simulink model "snake_model"  (R2018a)
settings: Solver=FixedStepAuto  StartTime=0.0  StopTime=Tmax  FixedStep=0.001  RelTol=1e-3
values from neighbouring files (symbols this model uses):
  theta_max = min(theta_max, pi/2)    [find_sat.m]    (also in run_3D_simulation.m = find_sat(jointCtrl.shape, (snake.n-1)/2, jointCtrl.alpha))
undefined symbols (not defined in the file or in its folder): attCtrl, ctrlSettings, dragcoeff, guidance, jointCtrl, pp, snake, thrustAlloc, velCtrl, y_0
libraries: vrlib x1, sharedutil x1
settings Model: Creator=ilborlau  LastModifiedBy=12037

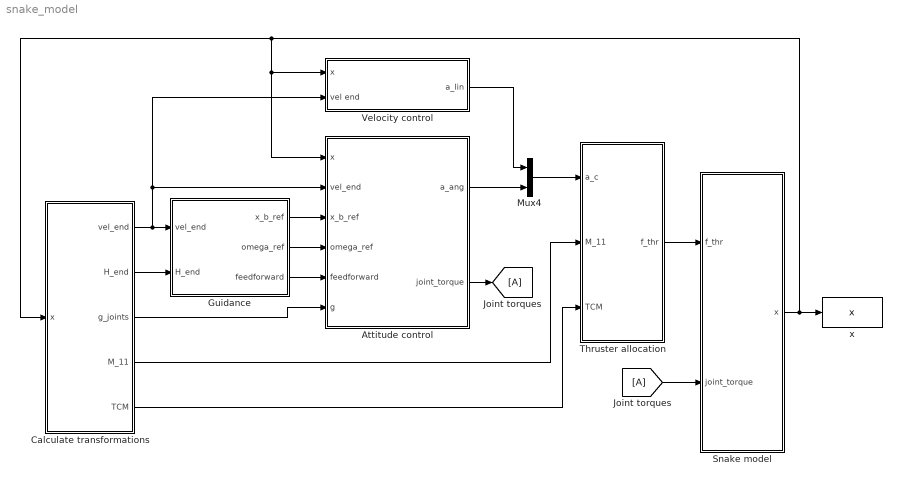
== system snake_model ==
  Attitude control : Subsystem
  Calculate transformations : Subsystem
  Guidance : Subsystem
  Mux4 : Mux  Inputs=2
  Snake model : Subsystem
  Thruster allocation : Subsystem
  Velocity control : Subsystem
  x : ToWorkspace  VariableName=x  SaveFormat=Structure With Time  SampleTime=-1
  wires:
  Guidance/1(x_b_ref) -> Attitude control/3(x_b_ref)
  [A] -> Snake model/2(joint_torque)
  Guidance/2(omega_ref) -> Attitude control/4(omega_ref)
  Guidance/3(feedforward) -> Attitude control/5(feedforward)
  Velocity control/1(a_lin) -> Mux4/1
  Attitude control/1("a_ang ") -> Mux4/2
  Calculate transformations/2(H_end) -> Guidance/2(H_end)
  Calculate transformations/1(vel_end) -> Guidance/1(vel_end), Velocity control/2(vel end), Attitude control/2(vel_end)
  Calculate transformations/5(TCM) -> Thruster allocation/3(TCM)
  Snake model/1(x) -> x/1, Calculate transformations/1(x), Velocity control/1(x), Attitude control/1(x)
  Thruster allocation/1(f_thr) -> Snake model/1(f_thr)
  Calculate transformations/4(M_11) -> Thruster allocation/2(M_11)
  Attitude control/2(joint_torque) -> [A]
  Calculate transformations/3(g_joints) -> Attitude control/6(g)
  Mux4/1 -> Thruster allocation/1(a_c)

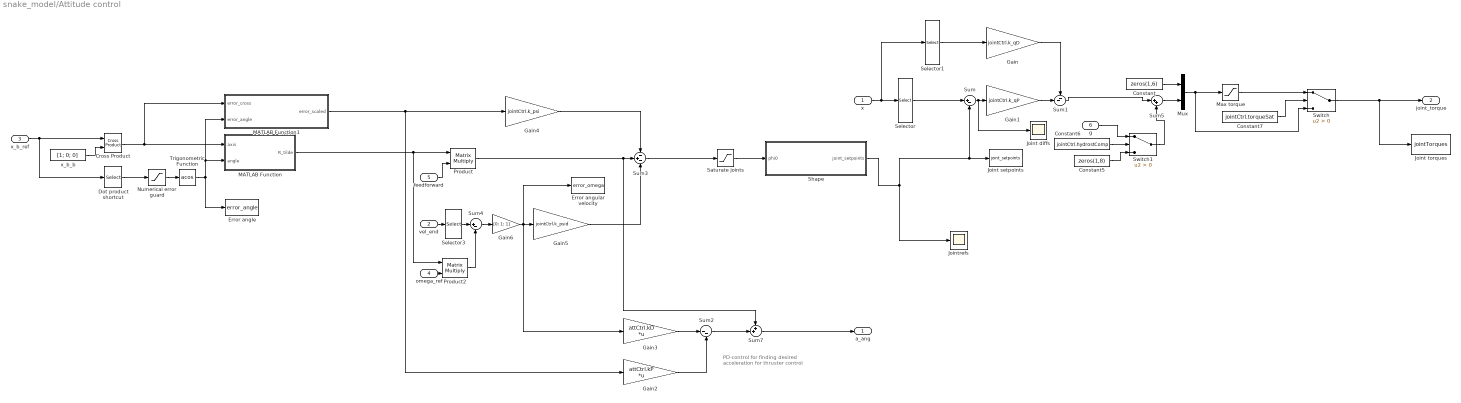
== system snake_model/Attitude control ==
  note: PD-control for finding desired acceleration for thruster control
  x : Inport
  vel_end : Inport  Port=2
  x_b_ref : Inport  Port=3
  omega_ref : Inport  Port=4
  feedforward : Inport  Port=5
  g : Inport  Port=6
  Constant : Constant  Value=zeros(1,6)
  Constant5 : Constant  Value=zeros(1,8)
  Constant6 : Constant  Value=jointCtrl.hydrostComp
  Constant7 : Constant  Value=jointCtrl.torqueSat
  Cross Product : vrlib/Utilities/Cross Product
      settings: SourceProductBaseCode=VR
  Dot product shortcut : Selector  InputPortWidth=3  IndexOptions=Index vector (dialog)  Indices=1  OutputSizes=1
  Error angle : ToWorkspace  VariableName=error_angle  SaveFormat=Structure With Time  SampleTime=-1
  Error angular velocity : ToWorkspace  VariableName=error_omega  SaveFormat=Structure With Time  SampleTime=-1
  Gain : Gain  Gain=jointCtrl.k_qD
  Gain1 : Gain  Gain=jointCtrl.k_qP
  Gain2 : Gain  Gain=attCtrl.kP  Multiplication=Matrix(K*u) (u vector)
  Gain3 : Gain  Gain=attCtrl.kD  Multiplication=Matrix(K*u) (u vector)
  Gain4 : Gain  Gain=jointCtrl.k_psi
  Gain5 : Gain  Gain=jointCtrl.k_psid
  Gain6 : Gain  Gain=[0; 1; 1]
  Joint diffs : Scope
  Joint setpoints : ToWorkspace  VariableName=joint_setpoints  SaveFormat=Structure With Time  SampleTime=-1
  Joint torques : ToWorkspace  VariableName=jointTorques  SaveFormat=Structure With Time  SampleTime=-1
  Jointrefs : Scope
  MATLAB Function : MATLAB Function  TreatAsAtomicUnit=on
  MATLAB Function1 : MATLAB Function  TreatAsAtomicUnit=on
  Max torque : Saturate  UpperLimit=11  LowerLimit=-11
  Mux : Mux  Inputs=2
  Numerical error guard : Saturate  UpperLimit=1  LowerLimit=-1
  Product : Product  Multiplication=Matrix(*)
  Product2 : Product  Multiplication=Matrix(*)
  Saturate joints : Saturate  UpperLimit=theta_max  LowerLimit=-theta_max
  Selector : Selector  InputPortWidth=11+2*snake.n  IndexOptions=Index vector (dialog)  Indices=8:6+snake.n  OutputSizes=1
  Selector1 : Selector  InputPortWidth=11+2*snake.n  IndexOptions=Index vector (dialog)  Indices=13+snake.n:11+2*snake.n  OutputSizes=1
  Selector3 : Selector  InputPortWidth=6  IndexOptions=Index vector (dialog)  Indices=4:6  OutputSizes=1
  Shape : MATLAB Function  TreatAsAtomicUnit=on
  Sum : Sum  Inputs=|+-
  Sum1 : Sum  Inputs=--|
  Sum2 : Sum  Inputs=|--
  Sum3 : Sum  Inputs=-+-
  Sum4 : Sum  Inputs=|+-
  Sum5 : Sum  Inputs=|++
  Sum7 : Sum  Inputs=++|
  Switch : Switch  Criteria=u2 > Threshold
  Switch1 : Switch  Criteria=u2 > Threshold
  Trigonometric Function : Trigonometry  Operator=acos
  x_b_b : Constant  Value=[1; 0; 0]
  "a_ang " : Outport
  joint_torque : Outport  Port=2
  wires:
  x_b_ref/1 -> Dot product shortcut/1, Cross Product/1
  omega_ref/1 -> Product2/2
  x/1 -> Selector1/1, Selector/1
  Sum/1 -> Joint diffs/1, Gain1/1
  Selector/1 -> Sum/1
  Gain1/1 -> Sum1/2
  Gain/1 -> Sum1/1
  Mux/1 -> Max torque/1, Switch/3
  Constant/1 -> Mux/1
  Shape/1(joint_setpoints) -> Sum/2, Joint setpoints/1, Jointrefs/1
  Gain3/1 -> Sum2/1
  Gain2/1 -> Sum2/2
  Sum2/1 -> Sum7/2
  x_b_b/1 -> Cross Product/2
  Cross Product/1 -> MATLAB Function/1(axis), MATLAB Function1/1(error_cross)
  vel_end/1 -> Selector3/1
  Selector3/1 -> Sum4/1
  MATLAB Function/1(R_tilde) -> Product/1, Product2/1
  feedforward/1 -> Product/2
  Sum4/1 -> Gain6/1
  Product2/1 -> Sum4/2
  Gain5/1 -> Sum3/3
  Gain4/1 -> Sum3/1
  Sum3/1 -> Saturate joints/1
  MATLAB Function1/1(error_scaled) -> Gain4/1, Gain2/1
  Selector1/1 -> Gain/1
  Dot product shortcut/1 -> Numerical error guard/1
  Numerical error guard/1 -> Trigonometric Function/1
  Trigonometric Function/1 -> Error angle/1, MATLAB Function1/2(error_angle), MATLAB Function/2(angle)
  Saturate joints/1 -> Shape/1(phi0)
  Switch/1 -> Joint torques/1, joint_torque/1
  Sum1/1 -> Sum5/1
  Sum7/1 -> "a_ang "/1
  Max torque/1 -> Switch/1
  Sum5/1 -> Mux/2
  Constant5/1 -> Switch1/3
  g/1 -> Switch1/1
  Constant6/1 -> Switch1/2
  Switch1/1 -> Sum5/2
  Constant7/1 -> Switch/2
  Product/1 -> Sum7/1, Sum3/2
  Gain6/1 -> Error angular velocity/1, Gain5/1, Gain3/1

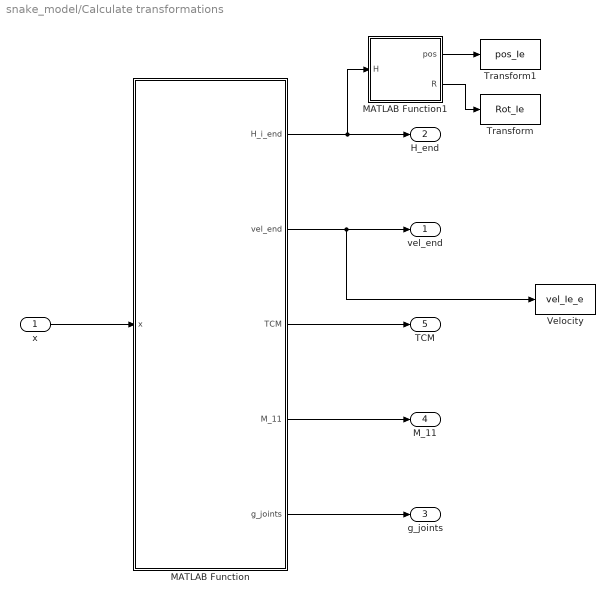
== system snake_model/Calculate transformations ==
  x : Inport
  MATLAB Function : MATLAB Function  TreatAsAtomicUnit=on
  MATLAB Function1 : MATLAB Function  TreatAsAtomicUnit=on
  Transform : ToWorkspace  VariableName=Rot_Ie  SaveFormat=Structure With Time  SampleTime=-1
  Transform1 : ToWorkspace  VariableName=pos_Ie  SaveFormat=Structure With Time  SampleTime=-1
  Velocity : ToWorkspace  VariableName=vel_Ie_e  SaveFormat=Structure With Time  SampleTime=-1
  vel_end : Outport
  H_end : Outport  Port=2
  g_joints : Outport  Port=3
  M_11 : Outport  Port=4
  TCM : Outport  Port=5
  wires:
  x/1 -> MATLAB Function/1(x)
  MATLAB Function/1(H_i_end) -> MATLAB Function1/1(H), H_end/1
  MATLAB Function/3(TCM) -> TCM/1
  MATLAB Function/2(vel_end) -> vel_end/1, Velocity/1
  MATLAB Function1/2(R) -> Transform/1
  MATLAB Function1/1(pos) -> Transform1/1
  MATLAB Function/5(g_joints) -> g_joints/1
  MATLAB Function/4(M_11) -> M_11/1

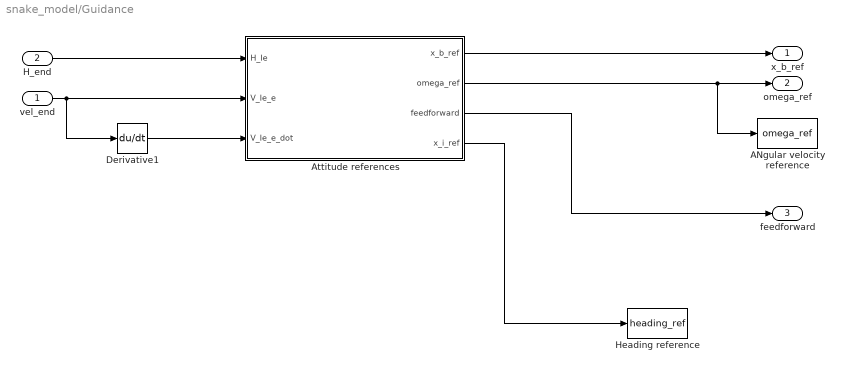
== system snake_model/Guidance ==
  vel_end : Inport
  H_end : Inport  Port=2
  ANgular velocity reference : ToWorkspace  VariableName=omega_ref  SaveFormat=Structure With Time  SampleTime=-1
  Attitude references : MATLAB Function  TreatAsAtomicUnit=on
  Derivative1 : Derivative  CoefficientInTFapproximation=1/15
  Heading reference : ToWorkspace  VariableName=heading_ref  SaveFormat=Structure With Time  SampleTime=-1
  x_b_ref : Outport
  omega_ref : Outport  Port=2
  feedforward : Outport  Port=3
  wires:
  H_end/1 -> Attitude references/1(H_Ie)
  Attitude references/1(x_b_ref) -> x_b_ref/1
  Attitude references/3(feedforward) -> feedforward/1
  Attitude references/4(x_i_ref) -> Heading reference/1
  vel_end/1 -> Derivative1/1, Attitude references/2(V_Ie_e)
  Attitude references/2(omega_ref) -> ANgular velocity reference/1, omega_ref/1
  Derivative1/1 -> Attitude references/3(V_Ie_e_dot)

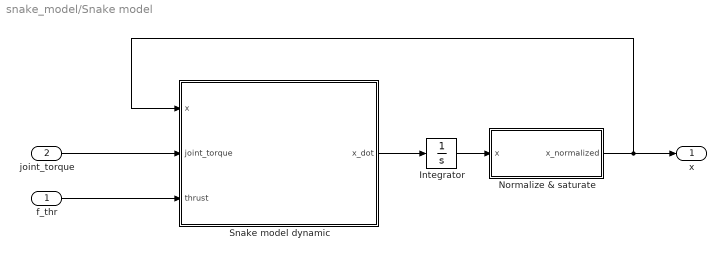
== system snake_model/Snake model ==
  f_thr : Inport
  joint_torque : Inport  Port=2
  Integrator : Integrator  InitialCondition=y_0
  Normalize & saturate : Subsystem
  Snake model dynamic : MATLAB Function  TreatAsAtomicUnit=on
  x : Outport
  wires:
  Snake model dynamic/1(x_dot) -> Integrator/1
  joint_torque/1 -> Snake model dynamic/2(joint_torque)
  f_thr/1 -> Snake model dynamic/3(thrust)
  Normalize & saturate/1(x_normalized) -> x/1, Snake model dynamic/1(x)
  Integrator/1 -> Normalize & saturate/1(x)

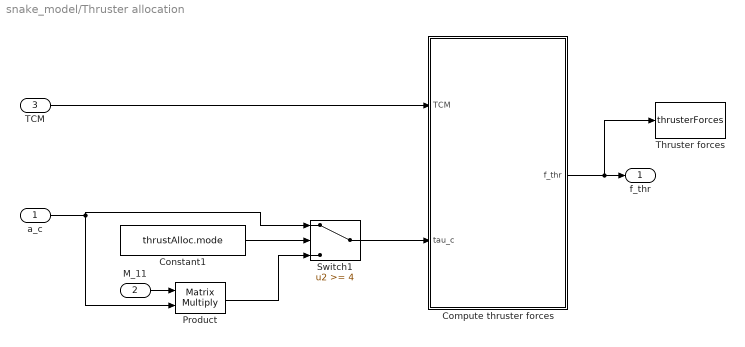
== system snake_model/Thruster allocation ==
  a_c : Inport
  M_11 : Inport  Port=2
  TCM : Inport  Port=3
  Compute thruster forces : MATLAB Function  TreatAsAtomicUnit=on
  Constant1 : Constant  Value=thrustAlloc.mode
  Product : Product  Multiplication=Matrix(*)
  Switch1 : Switch  Threshold=4
  Thruster forces : ToWorkspace  VariableName=thrusterForces  SaveFormat=Structure With Time  SampleTime=-1
  f_thr : Outport
  wires:
  TCM/1 -> Compute thruster forces/1(TCM)
  M_11/1 -> Product/1
  Constant1/1 -> Switch1/2
  Product/1 -> Switch1/3
  Switch1/1 -> Compute thruster forces/2(tau_c)
  a_c/1 -> Switch1/1, Product/2
  Compute thruster forces/1(f_thr) -> Thruster forces/1, f_thr/1

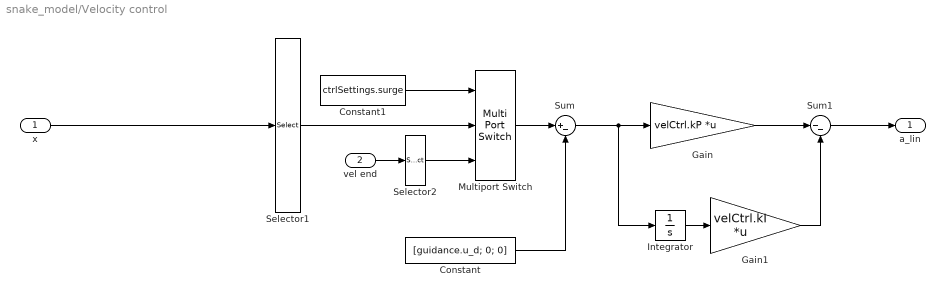
== system snake_model/Velocity control ==
  x : Inport
  vel end : Inport  Port=2
  Constant : Constant  Value=[guidance.u_d; 0; 0]
  Constant1 : Constant  Value=ctrlSettings.surge
  Gain : Gain  Gain=velCtrl.kP  Multiplication=Matrix(K*u) (u vector)
  Gain1 : Gain  Gain=velCtrl.kI  Multiplication=Matrix(K*u) (u vector)
  Integrator : Integrator
  Multiport Switch : MultiPortSwitch  DataPortOrder=Zero-based contiguous  Inputs=2  zeroidx=on
  Selector1 : Selector  InputPortWidth=11+2*snake.n  IndexOptions=Index vector (dialog)  Indices=7+snake.n:9+snake.n  OutputSizes=1
  Selector2 : Selector  InputPortWidth=6  IndexOptions=Index vector (dialog)  Indices=1:3  OutputSizes=1
  Sum : Sum  Inputs=|+-
  Sum1 : Sum  Inputs=|--
  a_lin : Outport
  wires:
  Selector1/1 -> Multiport Switch/2
  vel end/1 -> Selector2/1
  Multiport Switch/1 -> Sum/1
  Constant/1 -> Sum/2
  Sum/1 -> Integrator/1, Gain/1
  Integrator/1 -> Gain1/1
  Gain1/1 -> Sum1/2
  Gain/1 -> Sum1/1
  Selector2/1 -> Multiport Switch/3
  x/1 -> Selector1/1
  Sum1/1 -> a_lin/1
  Constant1/1 -> Multiport Switch/1

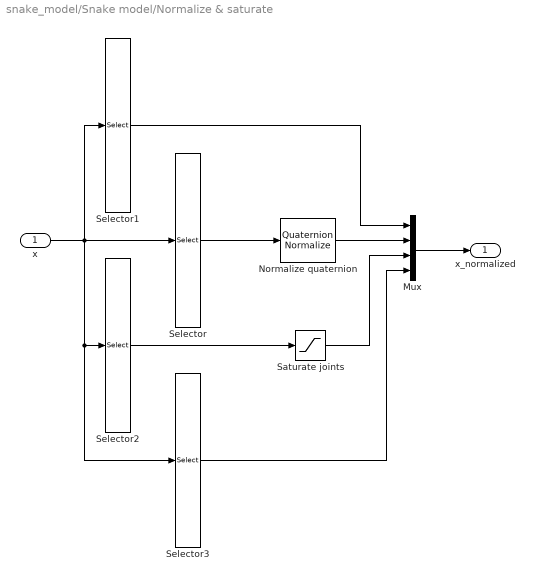
== system snake_model/Snake model/Normalize & saturate ==
  x : Inport
  Mux : Mux
  Normalize quaternion : sharedutil/Quaternion Normalize
      settings: SourceProductName=Aerospace Blockset  SourceProductBaseCode=AE
  Saturate joints : Saturate  UpperLimit=pi/2  LowerLimit=-pi/2
  Selector : Selector  InputPortWidth=11+2*snake.n  IndexOptions=Index vector (dialog)  Indices=4:7  OutputSizes=1
  Selector1 : Selector  InputPortWidth=11+2*snake.n  IndexOptions=Index vector (dialog)  Indices=1:3  OutputSizes=1
  Selector2 : Selector  InputPortWidth=11+2*snake.n  IndexOptions=Index vector (dialog)  Indices=8:6+snake.n  OutputSizes=1
  Selector3 : Selector  InputPortWidth=11+2*snake.n  IndexOptions=Index vector (dialog)  Indices=7+snake.n:11+2*snake.n  OutputSizes=1
  x_normalized : Outport
  wires:
  Mux/1 -> x_normalized/1
  x/1 -> Selector3/1, Selector2/1, Selector1/1, Selector/1
  Normalize quaternion/1 -> Mux/2
  Selector/1 -> Normalize quaternion/1
  Selector1/1 -> Mux/1
  Selector3/1 -> Mux/4
  Selector2/1 -> Saturate joints/1
  Saturate joints/1 -> Mux/3

== matlab function snake_model/Attitude control/Shape ==
  data: joint_setpoints output; phi0 input; jointCtrl parameter; snake parameter
function joint_setpoints  = generateJointSetpoints(phi0, jointCtrl, snake)
    
    %find indices of joints rotating about y- and z-axes
    y_joints = find(snake.joint_vec==2);
    z_joints = find(snake.joint_vec==3);
    
    switch jointCtrl.shape
        case 1
            y_vec = ones(1,length(y_joints));
            z_vec = ones(1,length(y_joints));
        case 2
            y_vec = (1/length(y_joints))*(length(y_joints):-1:1);
            z_vec = (1/length(z_joints))*(length(z_joints):-1:1);
        case 3
            y_vec = exp(-jointCtrl.alpha*(0:1:length(y_joints)-1));
            z_vec = exp(-jointCtrl.alpha*(0:1:length(z_joints)-1));
        case 4
            y_vec = zeros(1,length(y_joints));
            z_vec = zeros(1,length(y_joints));
            
        otherwise %case 1, uniform curve
            y_vec = ones(1,length(y_joints));
            z_vec = ones(1,length(y_joints));
    end
    
    joint_setpoints = zeros(size(snake.joint_vec))';
    joint_setpoints(y_joints) = phi0(2)*y_vec;
    joint_setpoints(z_joints) = phi0(3)*z_vec;

== matlab function snake_model/Snake model/Snake model dynamic ==
  data: x_dot output; x input; pp parameter; snake parameter; dragcoeff parameter; joint_torque input; thrust input
function x_dot  = dyn(x,pp, snake,dragcoeff,joint_torque,thrust)
x_dot = zeros(11+2*snake.n,1);

%Get states
pos       =  x(1:3);
quat      =  x(4:7);
theta     =  x(8 : 6+snake.n); %Joint angles
zeta      =  x(7+snake.n : 11+2*snake.n); %Body-velocities (6) + joint velocities

%Compute rotation matrices and jacobians
[R, J]    =  comp_rot_jac(quat,theta,snake);
%Compute mass matrix
M         =  comp_mass(J,snake);

%Compute relative velocity to take into account the effect of current
velc_h    =  R(:,:,1)'*pp.velc;
nu        =  zeta(1:6);
zeta(1:3) =  zeta(1:3)-velc_h;

%Compute coriolis, drag, and hydrostatic terms with the relative velocity
[c, d, g] =  comp_cdg(J,R,theta,snake,pp,dragcoeff,zeta);

%Compute the thrust-configuration matrix
B         =  comp_TCM(J,snake); %Number of thruster x 10 matrix, states + joints

%Compute the relative acceleration
zeta_dot      =  M\(B*thrust+joint_torque-c-d-g);

%Remove the effect of current
zeta_dot(1:3) = zeta_dot(1:3)-cross(nu(4:6),velc_h);
%Compute the time derivatives of position and orientation
pos_dot   =  R(:,:,1)*nu(1:3);
%pos_dot(3) = -pos_dot(3);
quat_dot  =  TransAngQ(quat)*nu(4:6)+1*(1-quat'*quat)*quat; 
%Assemble derivative of the state vector
%x_dot = [pos_dot ; quat_dot ; zeta(7:snake.n+5) ; zeta_dot];
x_dot(1:3) = pos_dot; %improved a little for speed by Marianna
x_dot(4:7) = quat_dot;
x_dot(8:6+snake.n) = zeta(7:snake.n+5);
x_dot(7+snake.n:11+2*snake.n) = zeta_dot;

end

== matlab function snake_model/Guidance/Attitude references ==
  data: H_Ie input; x_b_ref output; omega_ref output; feedforward output; x_i_ref output; guidance parameter; V_Ie_e input; V_Ie_e_dot input
function [x_b_ref, omega_ref, feedforward, x_i_ref]  = findAttitudeReferences(H_Ie, guidance, V_Ie_e, V_Ie_e_dot)
    % Finds the reference direction, reference angular velocity and
    % derivative of direction (for feedforward)
    R_Ie = H_Ie(1:3,1:3);
    p_Ie = H_Ie(1:3,4);
    
    if guidance.testMode == 1
% norm_inv_dot: 归一化项的导数，用于计算加速度和前馈控制。
% x_i_ref_dot:  归一化参考方向的导数，部分贡献于角速度。
% x_i_ref_ddot: 归一化参考方向的二阶导数，用于计算加速度。
       x_i_ref = guidance.constRef/norm(guidance.constRef);
       x_i_ref_dot = zeros(3,1);
       x_i_ref_ddot = zeros(3,1);
    else
        ref = [guidance.u_d; 0; 0] - guidance.k_cross*[0; p_Ie(2:3)]; %reference direction in path frame
        norm_inv = 1/norm(ref);
        x_i_ref = norm_inv*ref;
        
        
%计算横向速度，这是末端执行器速度在垂直于路径方向上的分量。
        cross_track_vel = diag([0 1 1])*R_Ie*V_Ie_e(1:3);
        
        norm_inv_dot = -guidance.k_cross*(norm_inv^3)*dot([0; p_Ie(2:3)], cross_track_vel); %derivative of normalising term, needed for acceleration/feedforward
        
        x_i_ref_dot = -guidance.k_cross*norm_inv*cross_track_vel; %strictly speaking only part of x_i_ref_dot contributing to angular velocity
        
        x_i_ref_ddot = -2*norm_inv_dot*guidance.k_cross*cross_track_vel + guidance.k_cross*norm_inv*diag([0 1 1])*R_Ie*(cross(V_Ie_e(4:6), V_Ie_e(1:3)) - V_Ie_e_dot(1:3));
        
        %x_i_ref_dot = - norm_inv*guidance.k_cross*cross_track_vel - dot(guidance.k_cross*[0; p_Ie(2:3)], guidance.k_cross*cross_track_vel)*(norm_inv^2)*x_i_ref;  
    end
% x_b_ref: 在基座或末端执行器框架中的归一化参考方向。
% omega_ref: 通过 x_b_ref 和其导数计算得到的期望角速度。
    x_b_ref = R_Ie'*x_i_ref; %normalized reference in head/end-effector frame
    omega_ref = cross(x_b_ref, R_Ie'*x_i_ref_dot);
    feedforward = R_Ie'*cross(x_i_ref, x_i_ref_ddot);
    
%     error = cross([1; 0; 0], ref_bod);
%     
%     %find derivative
%     if norm(error) == 0
%         R_tilde = eye(3); %because axang2rotm returns NaN if axis is zero
%     else
%         R_tilde = axang2rotm([-error' asin(min(norm(error),1))]); %rotation matrix rotating reference to body x-axis. min in case of numerical errors
%     end
%     
%     ref_bod_d = -cross(V_Ie_e(4:6), ref_bod) - guidance.k_cross*(1/norm(ref_path))*R_Ie'*[0; V_Ie_e(2); V_Ie_e(3)]; %parts of derivative of the reference contributing to angular velocity
%     
%     omega_ref = R_tilde*cross(ref_bod, ref_bod_d);
%     
%     omega_err = V_Ie_e(4:6) - omega_ref;
    
    % for plotting later
    %x_i_ref = ref_path/norm(ref_path);

== matlab function snake_model/Thruster allocation/Compute thruster forces ==
  data: TCM input; tau_c input; snake parameter; f_thr output size=7; thrustAlloc parameter
function f_thr = distributeThrusterForces(TCM, tau_c, snake,thrustAlloc)

Q_inv = thrustAlloc.Q_thr_inv;
mode = thrustAlloc.mode;

n_thr = snake.n_thruster_tot;


% Calculates the distribution of the thruster forces

switch mode
    case 0   % Standard damped inverse TCM
        [TCM_inv] = calculateTCMInverse(TCM, Q_inv);
        
        [f_thr] = calculateThrusterForces(TCM_inv, tau_c);
        
    case 1   % Thrust allocation with prioritized linear motion (DOF 1-3)
        [TCM_inv_linear,TCM_inv_angular] = calculateTCMInversePrioritized(TCM, Q_inv);
        
        %TCM_inv = [TCM_inv_linear, TCM_inv_angular];
        
        [f_thr] = calculateThrusterForcesPrioritized(TCM(1:3,:),TCM_inv_linear,TCM_inv_angular, tau_c, n_thr);
    
    case 2   % Thrust allocation with inverse TCM using SVD
        TCM_inv = calculateTCMInverseSVD(TCM,0.1);
        [f_thr] = calculateThrusterForces(TCM_inv, tau_c);
        
    case 3 % case 0 with longitudinal thrusters only
        toggle_thrusters = zeros(1,n_thr);
        toggle_thrusters(find(snake.thruster_ax==1)) = 1;
        TCM = TCM*diag(toggle_thrusters);
        [TCM_inv] = calculateTCMInverse(TCM, Q_inv);
        [f_thr] = calculateThrusterForces(TCM_inv, tau_c);
        
    case 4 % plain surge control using longitudinal thrusters
        f_thr = zeros(n_thr,1);
        for i = 1:n_thr
            if snake.thruster_ax(i) == 1  
                f_thr(i) = tau_c(1);
            end
        end
          
    otherwise  % Equal to case 0
        [TCM_inv] = calculateTCMInverse(TCM, Q_inv);
        
        [f_thr] = calculateThrusterForces(TCM_inv, tau_c);        
end

% saturate thruster forces

f_thr = min(max(f_thr, -40), 40);

end

== matlab function snake_model/Attitude control/MATLAB Function ==
  data: axis input; R_tilde output; angle input
function R_tilde = findErrorRotation(axis, angle)

    if norm(axis) == 0
        R_tilde = eye(3); %because axang2rotm returns NaN if axis is zero
    else
        R_tilde = axang2rotm([axis' angle]); %rotation matrix rotating reference to body x-axis
    end

== matlab function snake_model/Attitude control/MATLAB Function1 ==
  data: error_cross input size=3; error_scaled output size=3; error_angle input
function error_scaled = scaleByAngle(error_cross, error_angle)
    
    sin_theta = norm(error_cross);
    
    if sin_theta == 0 %avoid division by 0
        error_scaled = error_cross;
    else
        error_scaled = (error_angle/sin_theta)*error_cross;
    end

== matlab function snake_model/Calculate transformations/MATLAB Function ==
  data: x input; H_i_end output; vel_end output; TCM output; M_11 output; snake parameter; g_joints output; pp parameter; ctrlSettings parameter
function [H_i_end, vel_end, TCM, M_11, g_joints] = calculate_transforms(x, snake, pp, ctrlSettings)
    pos = x(1:3);
    quat = x(4:7);
%     提取关节角度theta和关节角速度zeta。
    theta = x(8:6+snake.n);
    zeta = x(7+snake.n:11+2*snake.n);
    
    % find transformation from inertial frame and base to end-effector
    H = [RotQ(quat) pos; 0 0 0 1]*A_HT(1,theta(1),snake);
    
    for i = 2:snake.n-1
        H = H*A_HT(i,theta(i),snake);
    end
    
    
    A_end = [eye(3) [snake.link(snake.n).length; 0; 0]; 0 0 0 1];
    H_i_end = H*A_end;
        
%计算旋转矩阵与旋转雅可比矩阵
    [R_base, J_base] = comp_rot_jac(quat,theta, snake);
    
    J_base_end = Ad_inv(A_end)*J_base(:,:,end);
    vel_end = J_base_end*zeta;
    
    
    %find "reverse" jacobians
    J_end = zeros(6,5+snake.n,snake.n);
    J_end(1:6,1:6,end) = Ad(A_end);
    
    for i = snake.n-1:-1:1
        A = A_HT(i,theta(i),snake);
        J_end(:,:,i) = Ad(A)*J_end(:,:,i+1);
        J_end(:,6+i,i) = -Ad(A)*snake.joint(i).twist;
    end
    
    if ctrlSettings.TCM %(1 is end-effector)
        TCM_full = comp_TCM(J_end, snake);
    else
        TCM_full = comp_TCM(J_base, snake);
    end
    
    %cut TCM's to thruster part only
    TCM = TCM_full(1:6,:);
    
    controlcase = 2*ctrlSettings.TCM + ctrlSettings.M_A; %the two take on values 1/0, so this gives four unique cases
    switch controlcase
        case 0 %TCM wrt base, rigid body
            M = J_base(:,:,1)'*snake.link(1).M_RB*J_base(:,:,1);
            for i = 2:snake.n
              M = M + J_base(:,:,i)'*snake.link(i).M_RB*J_base(:,:,i);
            end
        case 1 %base, added mass
            M = comp_mass(J_base, snake);
        case 2 %end-effector, RB
            M = J_end(:,:,1)'*snake.link(1).M_RB*J_end(:,:,1);
            for i = 2:snake.n
              M = M + J_end(:,:,i)'*snake.link(i).M_RB*J_end(:,:,i);
            end
        case 3 %end-effector, added mass
            M = comp_mass(J_end, snake);
    end
    
    M_11 = M(1:6,1:6);
    
    
    %taken from comp_cdg:
    g  = J_base(:,:,1)'*snake.link(1).G*R_base(:,:,1)'*pp.gdir;
    for i=2:snake.n
        g = g + J_base(:,:,i)'*snake.link(i).G*R_base(:,:,i)'*pp.gdir;
    end
    
    g_joints = g(7:end);

== matlab function snake_model/Calculate transformations/MATLAB Function1 ==
  data: H input; pos output; R output
function [pos, R] = extract(H)
R = H(1:3,1:3);
pos = H(1:3,4);
